simulink library "INT_AirCtl_CtlValCalc"  (R2016b)
settings: Solver=VariableStepAuto  StartTime=0.0  StopTime=10.0  RelTol=1e-3
settings Model: Creator=zhulinfeng  LastModifiedBy=zhulinfeng

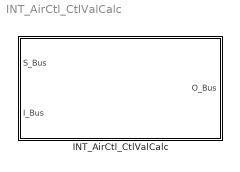
== system INT_AirCtl_CtlValCalc ==
  INT_AirCtl_CtlValCalc : Subsystem

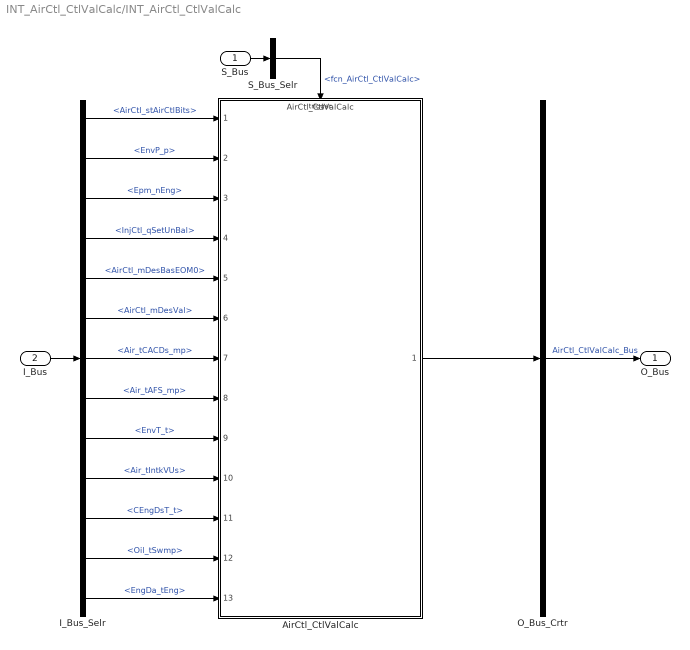
== system INT_AirCtl_CtlValCalc/INT_AirCtl_CtlValCalc ==
  S_Bus : Inport
  I_Bus : Inport  Port=2
  AirCtl_CtlValCalc : ModelReference  ModelNameDialog=AirCtl_CtlValCalc  SimulationMode=Normal  ModelReferenceVersion=1.17  TriggerPortName=function  TriggerPortTriggerType=function-call  TriggerPortStatesWhenEnabling=held
  I_Bus_Selr : BusSelector  OutputSignals=AirCtl_stAirCtlBits,EnvP_p,Epm_nEng,InjCtl_qSetUnBal,AirCtl_mDesBasEOM0,AirCtl_mDesVal,Air_tCACDs_mp,Air_tAFS_mp,EnvT_t,Air_tIntkVUs,CEngDsT_t,Oil_tSwmp,EngDa_tEng
  O_Bus_Crtr : BusCreator  Inputs=1
  S_Bus_Selr : BusSelector  OutputSignals=fcn_AirCtl_CtlValCalc
  O_Bus : Outport
  wires:
  S_Bus_Selr/1 -> AirCtl_CtlValCalc/Trigger  "<fcn_AirCtl_CtlValCalc>"
  S_Bus/1 -> S_Bus_Selr/1
  I_Bus/1 -> I_Bus_Selr/1
  I_Bus_Selr/1 -> AirCtl_CtlValCalc/1  "<AirCtl_stAirCtlBits>"
  I_Bus_Selr/2 -> AirCtl_CtlValCalc/2  "<EnvP_p>"
  I_Bus_Selr/3 -> AirCtl_CtlValCalc/3  "<Epm_nEng>"
  I_Bus_Selr/4 -> AirCtl_CtlValCalc/4  "<InjCtl_qSetUnBal>"
  I_Bus_Selr/5 -> AirCtl_CtlValCalc/5  "<AirCtl_mDesBasEOM0>"
  I_Bus_Selr/6 -> AirCtl_CtlValCalc/6  "<AirCtl_mDesVal>"
  I_Bus_Selr/7 -> AirCtl_CtlValCalc/7  "<Air_tCACDs_mp>"
  I_Bus_Selr/8 -> AirCtl_CtlValCalc/8  "<Air_tAFS_mp>"
  I_Bus_Selr/9 -> AirCtl_CtlValCalc/9  "<EnvT_t>"
  I_Bus_Selr/10 -> AirCtl_CtlValCalc/10  "<Air_tIntkVUs>"
  I_Bus_Selr/11 -> AirCtl_CtlValCalc/11  "<CEngDsT_t>"
  I_Bus_Selr/12 -> AirCtl_CtlValCalc/12  "<Oil_tSwmp>"
  I_Bus_Selr/13 -> AirCtl_CtlValCalc/13  "<EngDa_tEng>"
  O_Bus_Crtr/1 -> O_Bus/1  "AirCtl_CtlValCalc_Bus"
  AirCtl_CtlValCalc/1 -> O_Bus_Crtr/1
